simulink model "sim_kalman01"  (R2015a)
settings: Solver=ode45  StartTime=0.0  StopTime=9  FixedStep=1  MaxStep=1  RelTol=1e-3
undefined symbols (not defined in the file or in its folder): Discrete, Time
libraries: ctrlSharedLib x1
settings Model: Creator=liuqi  LastModifiedBy=liuqi

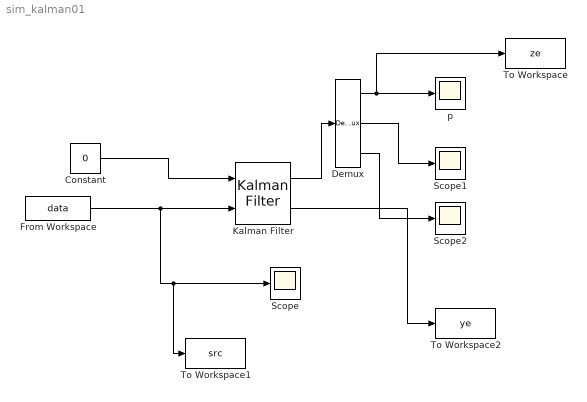
== system sim_kalman01 ==
  Constant : Constant  Value=0
  Demux : Demux  Outputs=3
  From Workspace : FromWorkspace  VariableName=data  SampleTime=1  Interpolate=off  OutputAfterFinalValue=Setting to zero
  Kalman Filter : ctrlSharedLib/Kalman Filter  TimeDomain=Discrete-Time  UseCurrentEstimator=on  ModelSource=Individual A, B, C, D matrices  ModelSourceVariable=ss(0.95,1,1,0,1)  A=[1, 0.1, 0.005; 0, 1, 0.1; 0, 0, 1]  B=[0;0;0]  C=[1, 0, 0; 1, 0, 0]  D=0  NumberOfStates=1  NumberOfInputs=1  NumberOfOutputs=1  InitialEstimateSource=Dialog  X0=0  P0=10  UseK=off  UseGH=off  NumberOfProcessNoiseInputs=1  G=1  TimeInvariantG=on  H=0  TimeInvariantH=on  Q=[0.5, 0, 0; 0, 0.01, 0; 0, 0, 0.001]  TimeInvariantQ=on  R=[10, 0; 0, 9]  TimeInvariantR=on  N=0  TimeInvariantN=on  AddInputPort=on  AddEnablePort=off  ExternalReset=none  OutputEstimatedY=on  OutputP=off  Ts=1
  Scope : Scope
      settings: SaveName=ScopeData3
  Scope1 : Scope
      settings: ShowLegends=on
  Scope2 : Scope
      settings: ShowLegends=on  SaveName=ScopeData2
  To Workspace : ToWorkspace  VariableName=ze  SaveFormat=Structure With Time  SampleTime=-1
  To Workspace1 : ToWorkspace  VariableName=src  SaveFormat=Structure With Time  SampleTime=-1
  To Workspace2 : ToWorkspace  VariableName=ye  SaveFormat=Structure With Time  SampleTime=-1
  p : Scope
      settings: ShowLegends=on
  wires:
  From Workspace/1 -> Scope/1, To Workspace1/1, Kalman Filter/2
  Constant/1 -> Kalman Filter/1
  Kalman Filter/1 -> Demux/1
  Demux/1 -> To Workspace/1, p/1
  Demux/2 -> Scope1/1
  Demux/3 -> Scope2/1
  Kalman Filter/2 -> To Workspace2/1
